simulink model "Clutchless_P2_Parallel_ETE"  (R2017b)
settings: Solver=FixedStepAuto  StartTime=0.0  StopTime=length(Speed)  FixedStep=0.01  MaxStep=0.01  RelTol=1e-3  EnableMultiTasking=on
PostLoadFcn:
  | , if any(exist('dsrtsu_mdlpostloadfcn', 'file') == [2, 3, 6]), try dsrtsu_mdlpostloadfcn('Execute', bdroot); catch fprintf('Error in PostLoadFcn (dsrtsu_mdlpostloadfcn) for model "%s":\n %s\n', bdroot, lasterr); end, end,
undefined symbols (not defined in the file): ABSEnable, Actuators, air, APP1_OOR, APP2_OOR, APP_Mismatch, Brk_Flt, cal, ClutchEngag, Clutchless_HSC_ETE, CS_On_Control, Driver, eng, Engine, EngOverTemp, ENGTRQ_MSMCH_Degraded_CP, ENGTRQ_MSMCH_ErrCritical_CP, ENGTRQ_MSMCH_LimpHome_CP, EngTrqMismatch, env, ess, ESSOverTemp, gb, KeyPos_Flt, KeyPosition, lib_Actuators, lib_Clutchless_HSC_ETE, lib_Driver, lib_EMachine_2017a, lib_Sensors_2017a, LossCAN, Machine, max_vehicle_rad_air_flow, MCUOverTemp, mot, MotDirMismatch, MotOverTemp, MotTrqMismatch, mph2ms, PRNDL_Flt, RegenBrkDisable, RegenFault, Sensors, ShiftLeverPosition, Speed, SW_CS_ON, SW_Engine_ON, t_amb, time, tloop
libraries: simulink x97, Pneumatic_lib x11, nesl_utility x9, EC2_libraries x7, powerlib_meascontrol x2, CalculationGallon x1, lib_Chassis x1, lib_DCDC x1, lib_Differential x1, lib_HVESS x1, fl_lib x1, lib_OBC x1
(part 7 of 9)

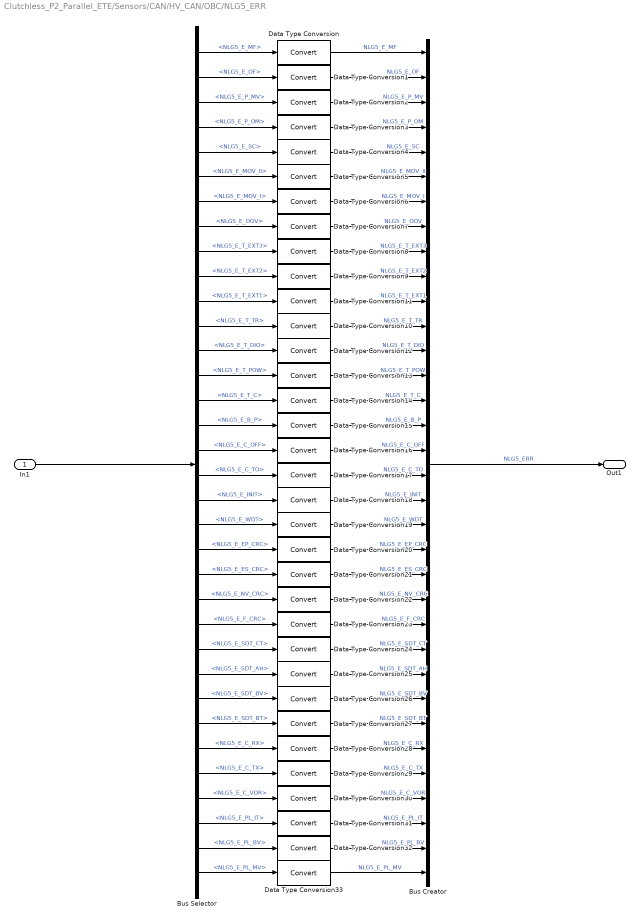
== system Clutchless_P2_Parallel_ETE/Sensors/CAN/HV_CAN/OBC/NLG5_ERR ==
  In1 : Inport
  Bus Creator : BusCreator  Inputs=34
  Bus Selector : BusSelector  OutputSignals=NLG5_E_MF,NLG5_E_OF,NLG5_E_P_MV,NLG5_E_P_OM,NLG5_E_SC,NLG5_E_MOV_II,NLG5_E_MOV_I,NLG5_E_OOV,NLG5_E_T_EXT3,NLG5_E_T_EXT2,NLG5_E_T_EXT1,NLG5_E_T_TR,NLG5_E_T_DIO,NLG5_E_T_POW,NLG5_E_T_C,NLG5_E_B_P,NLG5_E_C_OFF,NLG5_E_C_TO,NLG5_E_INIT,NLG5_E_WDT,NLG5_E_EP_CRC,NLG5_E_ES_CRC,NLG5_E_NV_CRC,NLG5_E_F_CRC,NLG5_E_SDT_CT,NLG5_E_SDT_AH,NLG5_E_SDT_BV,NLG5_E_SDT_BT,NLG5_E_C_RX,NLG5_E_C_TX,NLG5_E_C_VOR,NLG5_E_PL_IT,NLG5_E_PL_BV,NLG5_E_PL_MV
  Data Type Conversion{,1..33} (34 alike) : DataTypeConversion
  Out1 : Outport
  wires:
  Data Type Conversion4/1 -> Bus Creator/5  "NLG5_E_SC"
  Bus Selector/5 -> Data Type Conversion4/1  "<NLG5_E_SC>"
  In1/1 -> Bus Selector/1
  Bus Selector/1 -> Data Type Conversion/1  "<NLG5_E_MF>"
  Bus Selector/2 -> Data Type Conversion1/1  "<NLG5_E_OF>"
  Bus Selector/3 -> Data Type Conversion2/1  "<NLG5_E_P_MV>"
  Bus Selector/4 -> Data Type Conversion3/1  "<NLG5_E_P_OM>"
  Data Type Conversion/1 -> Bus Creator/1  "NLG5_E_MF"
  Data Type Conversion1/1 -> Bus Creator/2  "NLG5_E_OF"
  Data Type Conversion2/1 -> Bus Creator/3  "NLG5_E_P_MV"
  Data Type Conversion3/1 -> Bus Creator/4  "NLG5_E_P_OM"
  Bus Creator/1 -> Out1/1  "NLG5_ERR"
  Bus Selector/6 -> Data Type Conversion5/1  "<NLG5_E_MOV_II>"
  Bus Selector/34 -> Data Type Conversion33/1  "<NLG5_E_PL_MV>"
  Bus Selector/33 -> Data Type Conversion32/1  "<NLG5_E_PL_BV>"
  Bus Selector/32 -> Data Type Conversion31/1  "<NLG5_E_PL_IT>"
  Bus Selector/31 -> Data Type Conversion30/1  "<NLG5_E_C_VOR>"
  Bus Selector/30 -> Data Type Conversion29/1  "<NLG5_E_C_TX>"
  Bus Selector/29 -> Data Type Conversion28/1  "<NLG5_E_C_RX>"
  Bus Selector/28 -> Data Type Conversion27/1  "<NLG5_E_SDT_BT>"
  Bus Selector/27 -> Data Type Conversion26/1  "<NLG5_E_SDT_BV>"
  Bus Selector/7 -> Data Type Conversion6/1  "<NLG5_E_MOV_I>"
  Bus Selector/8 -> Data Type Conversion7/1  "<NLG5_E_OOV>"
  Bus Selector/9 -> Data Type Conversion8/1  "<NLG5_E_T_EXT3>"
  Bus Selector/10 -> Data Type Conversion9/1  "<NLG5_E_T_EXT2>"
  Bus Selector/11 -> Data Type Conversion11/1  "<NLG5_E_T_EXT1>"
  Bus Selector/12 -> Data Type Conversion10/1  "<NLG5_E_T_TR>"
  Bus Selector/13 -> Data Type Conversion12/1  "<NLG5_E_T_DIO>"
  Bus Selector/14 -> Data Type Conversion13/1  "<NLG5_E_T_POW>"
  Bus Selector/15 -> Data Type Conversion14/1  "<NLG5_E_T_C>"
  Bus Selector/16 -> Data Type Conversion15/1  "<NLG5_E_B_P>"
  Bus Selector/17 -> Data Type Conversion16/1  "<NLG5_E_C_OFF>"
  Bus Selector/18 -> Data Type Conversion17/1  "<NLG5_E_C_TO>"
  Bus Selector/19 -> Data Type Conversion18/1  "<NLG5_E_INIT>"
  Bus Selector/20 -> Data Type Conversion19/1  "<NLG5_E_WDT>"
  Bus Selector/21 -> Data Type Conversion20/1  "<NLG5_E_EP_CRC>"
  Bus Selector/22 -> Data Type Conversion21/1  "<NLG5_E_ES_CRC>"
  Bus Selector/23 -> Data Type Conversion22/1  "<NLG5_E_NV_CRC>"
  Bus Selector/24 -> Data Type Conversion23/1  "<NLG5_E_F_CRC>"
  Bus Selector/25 -> Data Type Conversion24/1  "<NLG5_E_SDT_CT>"
  Bus Selector/26 -> Data Type Conversion25/1  "<NLG5_E_SDT_AH>"
  Data Type Conversion5/1 -> Bus Creator/6  "NLG5_E_MOV_II"
  Data Type Conversion6/1 -> Bus Creator/7  "NLG5_E_MOV_I"
  Data Type Conversion7/1 -> Bus Creator/8  "NLG5_E_OOV"
  Data Type Conversion8/1 -> Bus Creator/9  "NLG5_E_T_EXT3"
  Data Type Conversion9/1 -> Bus Creator/10  "NLG5_E_T_EXT2"
  Data Type Conversion11/1 -> Bus Creator/11  "NLG5_E_T_EXT1"
  Data Type Conversion10/1 -> Bus Creator/12  "NLG5_E_T_TR"
  Data Type Conversion12/1 -> Bus Creator/13  "NLG5_E_T_DIO"
  Data Type Conversion13/1 -> Bus Creator/14  "NLG5_E_T_POW"
  Data Type Conversion14/1 -> Bus Creator/15  "NLG5_E_T_C"
  Data Type Conversion15/1 -> Bus Creator/16  "NLG5_E_B_P"
  Data Type Conversion16/1 -> Bus Creator/17  "NLG5_E_C_OFF"
  Data Type Conversion17/1 -> Bus Creator/18  "NLG5_E_C_TO"
  Data Type Conversion18/1 -> Bus Creator/19  "NLG5_E_INIT"
  Data Type Conversion19/1 -> Bus Creator/20  "NLG5_E_WDT"
  Data Type Conversion20/1 -> Bus Creator/21  "NLG5_E_EP_CRC"
  Data Type Conversion21/1 -> Bus Creator/22  "NLG5_E_ES_CRC"
  Data Type Conversion22/1 -> Bus Creator/23  "NLG5_E_NV_CRC"
  Data Type Conversion23/1 -> Bus Creator/24  "NLG5_E_F_CRC"
  Data Type Conversion24/1 -> Bus Creator/25  "NLG5_E_SDT_CT"
  Data Type Conversion25/1 -> Bus Creator/26  "NLG5_E_SDT_AH"
  Data Type Conversion26/1 -> Bus Creator/27  "NLG5_E_SDT_BV"
  Data Type Conversion27/1 -> Bus Creator/28  "NLG5_E_SDT_BT"
  Data Type Conversion28/1 -> Bus Creator/29  "NLG5_E_C_RX"
  Data Type Conversion29/1 -> Bus Creator/30  "NLG5_E_C_TX"
  Data Type Conversion30/1 -> Bus Creator/31  "NLG5_E_C_VOR"
  Data Type Conversion31/1 -> Bus Creator/32  "NLG5_E_PL_IT"
  Data Type Conversion32/1 -> Bus Creator/33  "NLG5_E_PL_BV"
  Data Type Conversion33/1 -> Bus Creator/34  "NLG5_E_PL_MV"

== system Clutchless_P2_Parallel_ETE/Sensors/CAN/HV_CAN/OBC/NLG5_ST ==
  In1 : Inport
  Bus Creator : BusCreator  Inputs=24
  Bus Selector : BusSelector  OutputSignals=NLG5_S_CP_DT,NLG5_S_UM_II,NLG5_S_UM_I,NLG5_S_EUM,NLG5_S_FAN,NLG5_S_WAR,NLG5_S_ERR,NLG5_S_HE,NLG5_S_L_PMAX,NLG5_S_L_CP,NLG5_S_L_PI,NLG5_S_L_MC,NLG5_S_L_OC,NLG5_S_L_OV,NLG5_S_BPD_II,NLG5_S_BPD_I,NLG5_S_L_T_BATT,NLG5_S_L_T_TR,NLG5_S_L_T_DIO,NLG5_S_L_T_POW,NLG5_S_L_T_CPRIM,NLG5_S_L_MO_MAX,NLG5_S_L_OC_MAX,NLG5_S_L_MC_MAX
  Data Type Conversion{,1..23} (24 alike) : DataTypeConversion
  Out1 : Outport
  wires:
  Data Type Conversion4/1 -> Bus Creator/5  "NLG5_S_FAN"
  Bus Selector/5 -> Data Type Conversion4/1  "<NLG5_S_FAN>"
  In1/1 -> Bus Selector/1
  Bus Selector/1 -> Data Type Conversion/1  "<NLG5_S_CP_DT>"
  Bus Selector/2 -> Data Type Conversion1/1  "<NLG5_S_UM_II>"
  Bus Selector/3 -> Data Type Conversion2/1  "<NLG5_S_UM_I>"
  Bus Selector/4 -> Data Type Conversion3/1  "<NLG5_S_EUM>"
  Data Type Conversion/1 -> Bus Creator/1  "NLG5_S_CP_DT"
  Data Type Conversion1/1 -> Bus Creator/2  "NLG5_S_UM_II"
  Data Type Conversion2/1 -> Bus Creator/3  "NLG5_S_UM_I"
  Data Type Conversion3/1 -> Bus Creator/4  "NLG5_S_EUM"
  Bus Creator/1 -> Out1/1  "NLG5_ST"
  Bus Selector/6 -> Data Type Conversion5/1  "<NLG5_S_WAR>"
  Bus Selector/7 -> Data Type Conversion6/1  "<NLG5_S_ERR>"
  Bus Selector/8 -> Data Type Conversion7/1  "<NLG5_S_HE>"
  Bus Selector/9 -> Data Type Conversion8/1  "<NLG5_S_L_PMAX>"
  Bus Selector/10 -> Data Type Conversion9/1  "<NLG5_S_L_CP>"
  Bus Selector/11 -> Data Type Conversion10/1  "<NLG5_S_L_PI>"
  Bus Selector/12 -> Data Type Conversion11/1  "<NLG5_S_L_MC>"
  Bus Selector/13 -> Data Type Conversion12/1  "<NLG5_S_L_OC>"
  Bus Selector/14 -> Data Type Conversion13/1  "<NLG5_S_L_OV>"
  Bus Selector/15 -> Data Type Conversion14/1  "<NLG5_S_BPD_II>"
  Bus Selector/16 -> Data Type Conversion15/1  "<NLG5_S_BPD_I>"
  Bus Selector/17 -> Data Type Conversion16/1  "<NLG5_S_L_T_BATT>"
  Bus Selector/18 -> Data Type Conversion17/1  "<NLG5_S_L_T_TR>"
  Bus Selector/19 -> Data Type Conversion18/1  "<NLG5_S_L_T_DIO>"
  Bus Selector/20 -> Data Type Conversion19/1  "<NLG5_S_L_T_POW>"
  Bus Selector/21 -> Data Type Conversion20/1  "<NLG5_S_L_T_CPRIM>"
  Bus Selector/22 -> Data Type Conversion21/1  "<NLG5_S_L_MO_MAX>"
  Bus Selector/23 -> Data Type Conversion22/1  "<NLG5_S_L_OC_MAX>"
  Bus Selector/24 -> Data Type Conversion23/1  "<NLG5_S_L_MC_MAX>"
  Data Type Conversion5/1 -> Bus Creator/6  "NLG5_S_WAR"
  Data Type Conversion7/1 -> Bus Creator/8  "NLG5_S_HE"
  Data Type Conversion6/1 -> Bus Creator/7  "NLG5_S_ERR"
  Data Type Conversion8/1 -> Bus Creator/9  "NLG5_S_L_PMAX"
  Data Type Conversion9/1 -> Bus Creator/10  "NLG5_S_L_CP"
  Data Type Conversion10/1 -> Bus Creator/11  "NLG5__S_L_PI"
  Data Type Conversion11/1 -> Bus Creator/12  "NLG5_S_L_MC"
  Data Type Conversion12/1 -> Bus Creator/13  "NLG5_S_L_OC"
  Data Type Conversion13/1 -> Bus Creator/14  "NLG5_S_L_OV"
  Data Type Conversion14/1 -> Bus Creator/15  "NLG5_S_BPD_II"
  Data Type Conversion15/1 -> Bus Creator/16  "NLG5_S_BPD_I"
  Data Type Conversion16/1 -> Bus Creator/17  "NLG5_S_L_T_BATT"
  Data Type Conversion17/1 -> Bus Creator/18  "NLG5_S_L_T_TR"
  Data Type Conversion18/1 -> Bus Creator/19  "NLG5_S_L_T_DIO"
  Data Type Conversion19/1 -> Bus Creator/20  "NLG5_S_L_T_POW"
  Data Type Conversion20/1 -> Bus Creator/21  "NLG5_S_L_T_CPRM"
  Data Type Conversion21/1 -> Bus Creator/22  "NLG5_S_L_MO_MAX"
  Data Type Conversion22/1 -> Bus Creator/23  "NLG5_S_L_OC_MAX"
  Data Type Conversion23/1 -> Bus Creator/24  "NLG5_S_L_MC_MAX"

== system Clutchless_P2_Parallel_ETE/Sensors/CAN/HV_CAN/OBC/NLG5_TEMP ==
  In1 : Inport
  Bus Creator : BusCreator  Inputs=4
  Bus Selector : BusSelector  OutputSignals=NLG5_P_TMP,NLG5_TMP_EXT1,NLG5_TMP_EXT2,NLG5_TMP_EXT3
  Data Type Conversion{,1..3} (4 alike) : DataTypeConversion
  Out1 : Outport
  wires:
  In1/1 -> Bus Selector/1
  Bus Selector/1 -> Data Type Conversion/1  "<NLG5_P_TMP>"
  Bus Selector/2 -> Data Type Conversion1/1  "<NLG5_TMP_EXT1>"
  Bus Selector/3 -> Data Type Conversion2/1  "<NLG5_TMP_EXT2>"
  Bus Selector/4 -> Data Type Conversion3/1  "<NLG5_TMP_EXT3>"
  Data Type Conversion/1 -> Bus Creator/1  "NLG5_P_TMP"
  Data Type Conversion1/1 -> Bus Creator/2  "NLG5_TMP_EXT1"
  Data Type Conversion2/1 -> Bus Creator/3  "NLG5_TMP_EXT2"
  Data Type Conversion3/1 -> Bus Creator/4  "NLG5_TMP_EXT3"
  Bus Creator/1 -> Out1/1  "NLG5_TEMP"

== system Clutchless_P2_Parallel_ETE/Sensors/CAN/VEH_CAN/BCM/PPEI_Brake_Apply_Status ==
  In1 : Inport
  Out1 : Outport
  wires:
  In1/1 -> Out1/1  "BrkPdlPos"

== system Clutchless_P2_Parallel_ETE/Sensors/CAN/VEH_CAN/BCM/PPEI_Platfrom_General_Status ==
  In1 : Inport
  Out1 : Outport
  wires:
  In1/1 -> Out1/1  "SysPwrMd"

== system Clutchless_P2_Parallel_ETE/Sensors/CAN/VEH_CAN/EBCM/PPEI_Chassis_General_Status_1 ==
  In1 : Inport
  Out1 : Outport
  wires:
  In1/1 -> Out1/1  "BrkPdlDrvAppPrsDetcd"

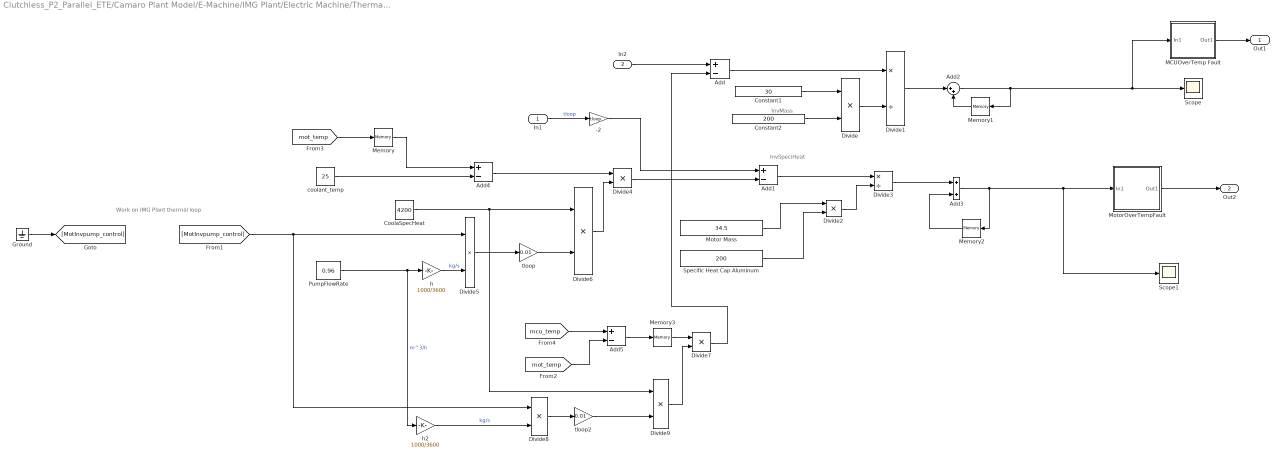
== system Clutchless_P2_Parallel_ETE/Camaro Plant Model/E-Machine/IMG Plant/Electric Machine/Thermal1/MotInv_loop ==
  note: Work on IMG Plant thermal loop
  note: InvMass
  note: InvSpeciHeat
  In1 : Inport
  In2 : Inport  Port=2
  -2 : Gain  Gain=tloop
  Add{,1,4..5} (4 alike) : Sum  Inputs=+-
  Add2 : Sum  Inputs=|++
  Add3 : Sum
  Constant1 : Constant  Value=30
  Constant2 : Constant  Value=200
  CoolaSpecHeat : Constant  Value=4200
  Divide{,2,4..9} (8 alike) : Product  Inputs=**
  Divide1 : Product  Inputs=*/
  Divide3 : Product  Inputs=*/
  Ground : Ground
  MCUOverTemp Fault : Subsystem
  Memory : Memory
  Memory1 : Memory  InitialCondition=25
  Memory2 : Memory  InitialCondition=25
  Memory3 : Memory
  Motor Mass : Constant  Value=34.5
  MotorOverTempFault : Subsystem
  PumpFlowRate : Constant  Value=0.96
  Scope : Scope
  Scope1 : Scope
  Specific Heat Cap Aluminum : Constant  Value=200
  coolant_temp : Constant  Value=25
  h : Gain  Gain=1000/3600
  h2 : Gain  Gain=1000/3600
  tloop : Gain  Gain=0.01
  tloop2 : Gain  Gain=0.01
  Out1 : Outport
  Out2 : Outport  Port=2
  wires:
  [MotInvpump_control] -> Divide8/1, Divide5/1
  -2/1 -> Add1/1
  In2/1 -> Add/1
  In1/1 -> -2/1  "tloop"
  [mot_temp] -> Add5/2
  [mcu_temp] -> Add5/1
  [mot_temp] -> Memory/1
  MotorOverTempFault/1(Out1) -> Out2/1
  MCUOverTemp Fault/1(Out1) -> Out1/1
  Memory3/1 -> Divide7/1
  Add5/1 -> Memory3/1
  Divide4/1 -> Add1/2
  tloop2/1 -> Divide9/2
  Divide8/1 -> tloop2/1
  Divide9/1 -> Divide7/2
  h2/1 -> Divide8/2  "kg/s"
  PumpFlowRate/1 -> h2/1, h/1  "m^3/h"
  CoolaSpecHeat/1 -> Divide9/1, Divide6/1
  tloop/1 -> Divide6/2
  h/1 -> Divide5/2  "kg/s"
  Divide7/1 -> Add/2
  Divide1/1 -> Add2/1
  Motor Mass/1 -> Divide2/1
  Constant2/1 -> Divide/2
  Divide2/1 -> Divide3/2
  Add2/1 -> Memory1/1, Scope/1, MCUOverTemp Fault/1(In1)
  Divide5/1 -> tloop/1
  Divide3/1 -> Add3/1
  Divide6/1 -> Divide4/2
  Add3/1 -> Memory2/1, MotorOverTempFault/1(In1), Scope1/1
  Add4/1 -> Divide4/1
  Memory2/1 -> Add3/2
  Add/1 -> Divide1/1
  Constant1/1 -> Divide/1
  Specific Heat Cap Aluminum/1 -> Divide2/2
  Divide/1 -> Divide1/2
  coolant_temp/1 -> Add4/2
  Memory1/1 -> Add2/2
  Add1/1 -> Divide3/1
  Memory/1 -> Add4/1
  Ground/1 -> [MotInvpump_control]

== system Clutchless_P2_Parallel_ETE/Camaro Plant Model/E-Machine/IMG Plant/Electric Machine/Thermal1/Motor Thermal ==
  In1 : Inport
  Add1 : Sum  Inputs=+-
  Add2 : Sum
  Divide : Product  Inputs=*/
  Lower Limit : Subsystem  mask{Lolimit=t_amb+20}
      mask prompts: Lolimit "Lower Limit"
  Memory1 : Memory
  Motor Mass : Constant  Value=mot.plant.init.motor_mass
  Product : Product  RndMeth=Zero
  "Pump " : Constant  Value=0
  Specific Heat Cap Aluminum : Constant  Value=mot.plant.init.specific_heat
  tloop : Gain  Gain=tloop
  Out1 : Outport
  wires:
  Add1/1 -> tloop/1
  In1/1 -> Add1/1
  "Pump "/1 -> Add1/2
  Motor Mass/1 -> Product/1  "kg"
  tloop/1 -> Divide/1  "J"
  Divide/1 -> Add2/1
  Lower Limit/1(Out1) -> Memory1/1, Out1/1
  Add2/1 -> Lower Limit/1(In1)
  Memory1/1 -> Add2/2
  Product/1 -> Divide/2
  Specific Heat Cap Aluminum/1 -> Product/2  "J/kg*K"

== system Clutchless_P2_Parallel_ETE/Camaro Plant Model/E-Machine/IMG Plant/Electric Machine/Torque Calculation1/electric machine filter ==
  trq : Inport
  Interval Test : simulink/Logic and Bit Operations/Interval Test  IntervalClosedRight=on  uplimit=0.5  IntervalClosedLeft=on  lowlimit=-0.5  OutDataTypeStr=boolean
  Switch : Switch  Threshold=0.5
  electric machine time response : TransferFcn  Denominator=[mot.plant.init.time_response 1]
  filtered : Outport
  wires:
  Switch/1 -> filtered/1
  trq/1 -> Switch/1, electric machine time response/1, Interval Test/1
  Interval Test/1 -> Switch/2
  electric machine time response/1 -> Switch/3

== system Clutchless_P2_Parallel_ETE/Camaro Plant Model/E-Machine/IMG Plant/Electric Machine/Torque Calculation1/max torque  ==
  cmd : Inport
  speed : Inport  Port=2
  Memory : Memory
  Peak trq max - Motoring : Lookup  InputValues=mot.plant.init.regen.trq_max.idx1_spd  Table=mot.plant.init.motor.trq_max.map  LookUpMeth=Interpolation-Use End Values  SaturateOnIntegerOverflow=on
  Peak trq max - Regen : Lookup  InputValues=mot.plant.init.regen.trq_max.idx1_spd  Table=mot.plant.init.regen.trq_max.map  LookUpMeth=Interpolation-Use End Values  SaturateOnIntegerOverflow=on
  Switch1 : Switch  SaturateOnIntegerOverflow=on
  rad/s  to RPM : Gain  Gain=30/pi
  max torque : Outport
  wires:
  Peak trq max - Regen/1 -> Switch1/3
  rad/s  to RPM/1 -> Memory/1
  Memory/1 -> Peak trq max - Regen/1, Peak trq max - Motoring/1
  Switch1/1 -> max torque/1
  cmd/1 -> Switch1/2
  speed/1 -> rad/s  to RPM/1
  Peak trq max - Motoring/1 -> Switch1/1

== system Clutchless_P2_Parallel_ETE/Camaro Plant Model/E-Machine/IMG Plant2/Thermal/Motor Thermal/Lower Limit ==
  In1 : Inport
  Constant3 : Constant  Value=Lolimit
  MinMax : MinMax  Function=max  Inputs=2
  Out1 : Outport
  wires:
  MinMax/1 -> Out1/1
  Constant3/1 -> MinMax/2
  In1/1 -> MinMax/1

== system Clutchless_P2_Parallel_ETE/Camaro Plant Model/E-Machine/IMG Plant2/Thermal1/MotInv_loop/MCUOverTemp Fault ==
  In1 : Inport
  Gain : Gain  Gain=3
  Switch : Switch  Threshold=1
  Out1 : Outport
  wires:
  Switch/1 -> Out1/1
  Gain/1 -> Switch/1
  [MCUOverTemp] -> Switch/2
  In1/1 -> Gain/1, Switch/3

== system Clutchless_P2_Parallel_ETE/Camaro Plant Model/E-Machine/IMG Plant2/Thermal1/MotInv_loop/MotorOverTempFault ==
  In1 : Inport
  Gain : Gain  Gain=2
  Switch1 : Switch  Threshold=1
  Out1 : Outport
  wires:
  Switch1/1 -> Out1/1
  Gain/1 -> Switch1/1
  [MotOverTemp] -> Switch1/2
  In1/1 -> Switch1/3, Gain/1

== system Clutchless_P2_Parallel_ETE/Camaro Plant Model/E-Machine/IMG Plant2/Thermal1/Motor Thermal/Lower Limit ==
  In1 : Inport
  Constant3 : Constant  Value=Lolimit
  MinMax : MinMax  Function=max  Inputs=2
  Out1 : Outport
  wires:
  MinMax/1 -> Out1/1
  Constant3/1 -> MinMax/2
  In1/1 -> MinMax/1

== system Clutchless_P2_Parallel_ETE/Camaro Plant Model/E-Machine/Soft MCU/Torque Calculation1/max torque /Divide by zero ==
  In1 : Inport
  Compare To Constant : simulink/Logic and Bit Operations/Compare To Constant  relop===  const=0  OutDataTypeStr=boolean
  Constant1 : Constant
  Switch2 : Switch  Criteria=u2 > Threshold
  Out1 : Outport
  wires:
  Constant1/1 -> Switch2/1
  Compare To Constant/1 -> Switch2/2
  In1/1 -> Switch2/3, Compare To Constant/1
  Switch2/1 -> Out1/1

== system Clutchless_P2_Parallel_ETE/Camaro Plant Model/E-Machine/Soft MCU/Torque Calculation1/max torque /Heat index ==
  note: Heat index calculation
  cont torque : Inport
  torque : Inport  Port=2
  Abs : Abs  SaturateOnIntegerOverflow=on
  Divide : Subsystem  mask(Divide){}
      mask Display: disp('Divide')
  Heat Energy Factor : Integrator  InitialCondition=-0.3  LimitOutput=on  UpperSaturationLimit=1  LowerSaturationLimit=-0.3
  Heating Constant : Gain  Gain=0.3/mot.plant.init.t_max_trq  SaturateOnIntegerOverflow=on  OutDataTypeStr=Inherit: Same as input  ParamDataTypeStr=Inherit: Same as input
  Saturation : Saturate  UpperLimit=1  LowerLimit=0
  Sum : Sum  Inputs=+-  SaturateOnIntegerOverflow=on  InputSameDT=on  OutDataTypeStr=Inherit: Same as first input
  motor inertia (Nms^2\rad)5 : Constant
  Heat index : Outport
  wires:
  cont torque/1 -> Divide/2(denominator)
  Abs/1 -> Sum/1
  Saturation/1 -> Heat index/1
  motor inertia (Nms^2\rad)5/1 -> Sum/2
  Divide/1(quotient) -> Abs/1
  Sum/1 -> Heating Constant/1
  Heating Constant/1 -> Heat Energy Factor/1
  Heat Energy Factor/1 -> Saturation/1
  torque/1 -> Divide/1(numerator)

== system Clutchless_P2_Parallel_ETE/Camaro Plant Model/E-Machine/Soft MCU/Torque Calculation2/max torque /Divide by zero ==
  In1 : Inport
  Compare To Constant : simulink/Logic and Bit Operations/Compare To Constant  relop===  const=0  OutDataTypeStr=boolean
  Constant1 : Constant
  Switch2 : Switch  Criteria=u2 > Threshold
  Out1 : Outport
  wires:
  Constant1/1 -> Switch2/1
  Compare To Constant/1 -> Switch2/2
  In1/1 -> Switch2/3, Compare To Constant/1
  Switch2/1 -> Out1/1

== system Clutchless_P2_Parallel_ETE/Camaro Plant Model/E-Machine/Soft MCU/Torque Calculation2/max torque /Heat index ==
  note: Heat index calculation
  cont torque : Inport
  torque : Inport  Port=2
  Abs : Abs  SaturateOnIntegerOverflow=on
  Divide : Subsystem  mask(Divide){}
      mask Display: disp('Divide')
  Heat Energy Factor : Integrator  InitialCondition=-0.3  LimitOutput=on  UpperSaturationLimit=1  LowerSaturationLimit=-0.3
  Heating Constant : Gain  Gain=0.3/mot.plant.init.t_max_trq  SaturateOnIntegerOverflow=on  OutDataTypeStr=Inherit: Same as input  ParamDataTypeStr=Inherit: Same as input
  Saturation : Saturate  UpperLimit=1  LowerLimit=0
  Sum : Sum  Inputs=+-  SaturateOnIntegerOverflow=on  InputSameDT=on  OutDataTypeStr=Inherit: Same as first input
  motor inertia (Nms^2\rad)5 : Constant
  Heat index : Outport
  wires:
  cont torque/1 -> Divide/2(denominator)
  Abs/1 -> Sum/1
  Saturation/1 -> Heat index/1
  motor inertia (Nms^2\rad)5/1 -> Sum/2
  Divide/1(quotient) -> Abs/1
  Sum/1 -> Heating Constant/1
  Heating Constant/1 -> Heat Energy Factor/1
  Heat Energy Factor/1 -> Saturation/1
  torque/1 -> Divide/1(numerator)

== system Clutchless_P2_Parallel_ETE/Camaro Plant Model/ICE Simple1/Engine Plant Modified/Core Engine/Core Engine1/Upstream States ==
  K Converter : nesl_utility/PS-Simulink Converter  PhysicalDomain=network_engine_domain  SubClassName=ps_output  LeftPortType=input  RightPortType=output  PseudoPeriodic=off  Frequencies=[]  Unit=K  AffineConversion=off
  Pa Converter : nesl_utility/PS-Simulink Converter  PhysicalDomain=network_engine_domain  SubClassName=ps_output  LeftPortType=input  RightPortType=output  PseudoPeriodic=off  Frequencies=[]  Unit=Pa  AffineConversion=off
  Pneumatic Absolute Reference : Pneumatic_lib/Pneumatic Elements/Pneumatic Absolute Reference
  Pneumatic Pressure & Temperature Sensor : Pneumatic_lib/Pneumatic Sensors/Pneumatic Pressure & Temperature Sensor
  A : PMIOPort  Port=1  Side=Left
  P (Pa) : Outport
  T (K) : Outport  Port=2
  wires:
  Pa Converter/1 -> P (Pa)/1
  K Converter/1 -> T (K)/1
  connections:
  Pneumatic Pressure & Temperature Sensor/RConn1 -- Pneumatic Absolute Reference/LConn1
  Pneumatic Pressure & Temperature Sensor/LConn1 -- A/RConn1
  K Converter/LConn1 -- Pneumatic Pressure & Temperature Sensor/RConn3
  Pneumatic Pressure & Temperature Sensor/RConn2 -- Pa Converter/LConn1

== system Clutchless_P2_Parallel_ETE/Camaro Plant Model/ICE Simple1/Engine Plant Modified/Core Engine/EngEfficiency1/Divide by Zero Fix ==
  Multiply : Inport
  Divide : Inport  Port=2
  Compare To Zero : simulink/Logic and Bit Operations/Compare To Zero  relop===  OutDataTypeStr=boolean
  Constant1 : Constant  Value=0
  Constant2 : Constant
  Product2 : Product  Inputs=/*  SaturateOnIntegerOverflow=on  InputSameDT=on  OutDataTypeStr=Inherit: Same as first input
  Switch : Switch  Threshold=1
  Switch1 : Switch  Threshold=1
  Output : Outport
  wires:
  Multiply/1 -> Product2/2
  Switch1/1 -> Output/1
  Constant1/1 -> Switch1/1
  Product2/1 -> Switch1/3
  Switch/1 -> Product2/1
  Divide/1 -> Switch/3, Compare To Zero/1
  Constant2/1 -> Switch/1
  Compare To Zero/1 -> Switch1/2, Switch/2

== system Clutchless_P2_Parallel_ETE/Camaro Plant Model/ICE Simple1/Engine Plant Modified/Core Engine/Intake Manifold1/Node Potential Sensor ==
  K Converter : nesl_utility/PS-Simulink Converter  PhysicalDomain=network_engine_domain  SubClassName=ps_output  LeftPortType=input  RightPortType=output  PseudoPeriodic=off  Frequencies=[]  Unit=K  AffineConversion=off
  K to C : Fcn  Expr=u(1)-273.15
  Pa Converter : nesl_utility/PS-Simulink Converter  PhysicalDomain=network_engine_domain  SubClassName=ps_output  LeftPortType=input  RightPortType=output  PseudoPeriodic=off  Frequencies=[]  Unit=Pa  AffineConversion=off
  Pa to KPa : Gain  Gain=0.001
  Pneumatic Absolute Reference : Pneumatic_lib/Pneumatic Elements/Pneumatic Absolute Reference
  Pneumatic Pressure & Temperature Sensor : Pneumatic_lib/Pneumatic Sensors/Pneumatic Pressure & Temperature Sensor
  A : PMIOPort  Port=1  Side=Left
  P (KPa) : Outport
  T (C) : Outport  Port=2
  wires:
  Pa Converter/1 -> Pa to KPa/1
  K Converter/1 -> K to C/1
  K to C/1 -> T (C)/1
  Pa to KPa/1 -> P (KPa)/1
  connections:
  Pneumatic Pressure & Temperature Sensor/RConn1 -- Pneumatic Absolute Reference/LConn1
  Pneumatic Pressure & Temperature Sensor/LConn1 -- A/RConn1
  K Converter/LConn1 -- Pneumatic Pressure & Temperature Sensor/RConn3
  Pneumatic Pressure & Temperature Sensor/RConn2 -- Pa Converter/LConn1

== system Clutchless_P2_Parallel_ETE/Clutchless_HSC_ETE/HSC/Camaro Fault Detection/Component Diagnostic/Engine Component Diagnostic/Override  engTrqCmd ==
  note: This subsystem is used to override the model value of a signal to a constant value
  note: Override Switch Subsystem
  In1 : Inport
  Constant : Constant  Value=50
  Multiport Switch : MultiPortSwitch  DataPortOrder=Zero-based contiguous  Inputs=2  zeroidx=on
  Signal Override Switch 0 = Use Model 1 = Use Constant : Constant
  Out1 : Outport
  wires:
  Signal Override Switch 0 = Use Model 1 = Use Constant/1 -> Multiport Switch/1
  In1/1 -> Multiport Switch/2
  Multiport Switch/1 -> Out1/1
  Constant/1 -> Multiport Switch/3

== system Clutchless_P2_Parallel_ETE/Clutchless_HSC_ETE/HSC/Camaro Fault Detection/Component Diagnostic/Engine Component Diagnostic/TorqMismatch Detection ==
  In1 : Inport
  In2 : Inport  Port=2
  In3 : Inport  Port=3
  Abs : Abs
  Add : Sum  Inputs=+-
  Bus Creator : BusCreator  Inputs=3
  Constant : Constant  Value=cal.ENGTRQ_MSMCH.ErrCritical_CP
  Constant1 : Constant  Value=50
  Constant2 : Constant  Value=cal.ENGTRQ_MSMCH.Degraded_CP
  Constant3 : Constant  Value=cal.ENGTRQ_MSMCH.LimpHome_CP
  Constant4 : Constant  Value=0
  Constant5 : Constant  Value=0
  Constant6 : Constant  Value=0
  Data Type Conversion : DataTypeConversion  OutDataTypeStr=boolean
  Data Type Conversion1 : DataTypeConversion  OutDataTypeStr=boolean
  Data Type Conversion2 : DataTypeConversion  OutDataTypeStr=boolean
  Relational Operator : RelationalOperator  OutDataTypeStr=boolean  RndMeth=Nearest
  Relational Operator1 : RelationalOperator  Operator=>  OutDataTypeStr=boolean  RndMeth=Nearest
  Relational Operator2 : RelationalOperator  Operator=>  OutDataTypeStr=boolean  RndMeth=Nearest
  Switch : Switch  Threshold=1
  Terminator{,1..3} (4 alike) : Terminator
  Unit Delay : UnitDelay  Commented=through  SampleTime=-1
  Unit Delay1 : UnitDelay  Commented=through  SampleTime=-1
  "Zero " : Constant  Value=0
  Eng_Torque_Mismch : Outport
  wires:
  Constant1/1 -> Terminator3/1
  In1/1 -> Unit Delay/1
  In2/1 -> Unit Delay1/1
  "Zero "/1 -> Switch/3
  In3/1 -> Switch/2
  Unit Delay/1 -> Add/1
  Constant/1 -> Relational Operator/2
  Add/1 -> Abs/1
  Relational Operator/1 -> Switch/1
  Switch/1 -> Relational Operator2/1, Relational Operator1/1, Terminator/1  "Eng_Torque_Mismch_Critical"
  Constant2/1 -> Relational Operator1/2
  Constant3/1 -> Relational Operator2/2
  Relational Operator1/1 -> Terminator1/1  "Eng_Torque_Mismch_Degrad"
  Relational Operator2/1 -> Terminator2/1  "Eng_Torque_Mismch_Limp"
  Bus Creator/1 -> Eng_Torque_Mismch/1
  Unit Delay1/1 -> Add/2
  Abs/1 -> Relational Operator/1
  Constant4/1 -> Data Type Conversion/1  "Eng_Torque_Mismch_Critical"
  Constant6/1 -> Data Type Conversion2/1  "Eng_Torque_Mismch_Limp"
  Constant5/1 -> Data Type Conversion1/1  "Eng_Torque_Mismch_Degrad"
  Data Type Conversion/1 -> Bus Creator/1  "Eng_Torque_Mismch_Critical"
  Data Type Conversion1/1 -> Bus Creator/2  "Eng_Torque_Mismch_Degrad"
  Data Type Conversion2/1 -> Bus Creator/3  "Eng_Torque_Mismch_Limp"

== system Clutchless_P2_Parallel_ETE/Clutchless_HSC_ETE/HSC/Camaro Fault Detection/Input Conversions/BMS_Conversions/Override  BMS_gdf 0_1 ==
  note: Override Switch Subsystem
  note: This subsystem is used to override the model value of a signal to a constant value
  In1 : Inport
  Multiport Switch : MultiPortSwitch  DataPortOrder=Zero-based contiguous  Inputs=2  zeroidx=on
  Override Value : Constant  Value=0  OutDataTypeStr=double
  Signal Override Switch 0 = Use Model 1 = Use Constant : Constant
  Out1 : Outport
  wires:
  Override Value/1 -> Multiport Switch/3
  Multiport Switch/1 -> Out1/1
  In1/1 -> Multiport Switch/2
  Signal Override Switch 0 = Use Model 1 = Use Constant/1 -> Multiport Switch/1

== system Clutchless_P2_Parallel_ETE/Clutchless_HSC_ETE/HSC/Camaro Fault Detection/Input Conversions/BMS_Conversions/Override  closeContactorsCmd ==
  note: This subsystem is used to override the model value of a signal to a constant value
  note: Override Switch Subsystem
  In1 : Inport
  Multiport Switch : MultiPortSwitch  DataPortOrder=Zero-based contiguous  Inputs=2  zeroidx=on
  Override Value : Constant  Value=0  OutDataTypeStr=double
  Signal Override Switch 0 = Use Model 1 = Use Constant : Constant  Value=0
  Out1 : Outport
  wires:
  Signal Override Switch 0 = Use Model 1 = Use Constant/1 -> Multiport Switch/1
  In1/1 -> Multiport Switch/2
  Multiport Switch/1 -> Out1/1
  Override Value/1 -> Multiport Switch/3

== system Clutchless_P2_Parallel_ETE/Clutchless_HSC_ETE/HSC/Camaro Fault Detection/Input Conversions/BMS_Conversions/Override  contactorsClsd ==
  note: This subsystem is used to override the model value of a signal to a constant value
  note: Override Switch Subsystem
  In1 : Inport
  Multiport Switch : MultiPortSwitch  DataPortOrder=Zero-based contiguous  Inputs=2  zeroidx=on
  Override Value : Constant  Value=0  OutDataTypeStr=double
  Signal Override Switch 0 = Use Model 1 = Use Constant : Constant  Value=0
  Out1 : Outport
  wires:
  Signal Override Switch 0 = Use Model 1 = Use Constant/1 -> Multiport Switch/1
  In1/1 -> Multiport Switch/2
  Multiport Switch/1 -> Out1/1
  Override Value/1 -> Multiport Switch/3

== system Clutchless_P2_Parallel_ETE/Clutchless_HSC_ETE/HSC/Camaro Fault Detection/Input Conversions/BMS_Conversions/Override  essCur_A ==
  note: Override Switch Subsystem
  note: This subsystem is used to override the model value of a signal to a constant value
  In1 : Inport
  Multiport Switch : MultiPortSwitch  DataPortOrder=Zero-based contiguous  Inputs=2  zeroidx=on
  Override Value : Constant  Value=0  OutDataTypeStr=double
  Signal Override Switch 0 = Use Model 1 = Use Constant : Constant  Value=0
  Out1 : Outport
  wires:
  Override Value/1 -> Multiport Switch/3
  Multiport Switch/1 -> Out1/1
  In1/1 -> Multiport Switch/2
  Signal Override Switch 0 = Use Model 1 = Use Constant/1 -> Multiport Switch/1

== system Clutchless_P2_Parallel_ETE/Clutchless_HSC_ETE/HSC/Camaro Fault Detection/Input Conversions/BMS_Conversions/Override  essSOC_0_1 ==
  note: This subsystem is used to override the model value of a signal to a constant value
  note: Override Switch Subsystem
  In1 : Inport
  Multiport Switch : MultiPortSwitch  DataPortOrder=Zero-based contiguous  Inputs=2  zeroidx=on
  Override Value : Constant  Value=0  OutDataTypeStr=double
  Signal Override Switch 0 = Use Model 1 = Use Constant : Constant  Value=0
  Out1 : Outport
  wires:
  Signal Override Switch 0 = Use Model 1 = Use Constant/1 -> Multiport Switch/1
  In1/1 -> Multiport Switch/2
  Multiport Switch/1 -> Out1/1
  Override Value/1 -> Multiport Switch/3

== system Clutchless_P2_Parallel_ETE/Clutchless_HSC_ETE/HSC/Camaro Fault Detection/Input Conversions/BMS_Conversions/Override  essTemp_C ==
  note: This subsystem is used to override the model value of a signal to a constant value
  note: Override Switch Subsystem
  In1 : Inport
  Multiport Switch : MultiPortSwitch  DataPortOrder=Zero-based contiguous  Inputs=2  zeroidx=on
  Override Value : Constant  Value=0  OutDataTypeStr=double
  Signal Override Switch 0 = Use Model 1 = Use Constant : Constant
  Out1 : Outport
  wires:
  Signal Override Switch 0 = Use Model 1 = Use Constant/1 -> Multiport Switch/1
  In1/1 -> Multiport Switch/2
  Multiport Switch/1 -> Out1/1
  Override Value/1 -> Multiport Switch/3

== system Clutchless_P2_Parallel_ETE/Clutchless_HSC_ETE/HSC/Camaro Fault Detection/Input Conversions/BMS_Conversions/Override  hvBattVolt_V ==
  note: This subsystem is used to override the model value of a signal to a constant value
  note: Override Switch Subsystem
  In1 : Inport
  Multiport Switch : MultiPortSwitch  DataPortOrder=Zero-based contiguous  Inputs=2  zeroidx=on
  Override Value : Constant  Value=0  OutDataTypeStr=double
  Signal Override Switch 0 = Use Model 1 = Use Constant : Constant  Value=0
  Out1 : Outport
  wires:
  Signal Override Switch 0 = Use Model 1 = Use Constant/1 -> Multiport Switch/1
  In1/1 -> Multiport Switch/2
  Multiport Switch/1 -> Out1/1
  Override Value/1 -> Multiport Switch/3

== system Clutchless_P2_Parallel_ETE/Clutchless_HSC_ETE/HSC/Camaro Fault Detection/Input Conversions/BMS_Conversions/Override  hvBusVolt_V ==
  note: Override Switch Subsystem
  note: This subsystem is used to override the model value of a signal to a constant value
  In1 : Inport
  Multiport Switch : MultiPortSwitch  DataPortOrder=Zero-based contiguous  Inputs=2  zeroidx=on
  Override Value : Constant  Value=0  OutDataTypeStr=double
  Signal Override Switch 0 = Use Model 1 = Use Constant : Constant  Value=0
  Out1 : Outport
  wires:
  Override Value/1 -> Multiport Switch/3
  Multiport Switch/1 -> Out1/1
  In1/1 -> Multiport Switch/2
  Signal Override Switch 0 = Use Model 1 = Use Constant/1 -> Multiport Switch/1

== system Clutchless_P2_Parallel_ETE/Clutchless_HSC_ETE/HSC/Camaro Fault Detection/Input Conversions/BMS_Conversions/Override  rollingAliveCnt [1_3] ==
  note: Override Switch Subsystem
  note: This subsystem is used to override the model value of a signal to a constant value
  In1 : Inport
  Multiport Switch : MultiPortSwitch  DataPortOrder=Zero-based contiguous  Inputs=2  zeroidx=on
  Override Value : Constant  Value=0  OutDataTypeStr=double
  Signal Override Switch 0 = Use Model 1 = Use Constant : Constant  Value=0
  Out1 : Outport
  wires:
  Override Value/1 -> Multiport Switch/3
  Multiport Switch/1 -> Out1/1
  In1/1 -> Multiport Switch/2
  Signal Override Switch 0 = Use Model 1 = Use Constant/1 -> Multiport Switch/1

== system Clutchless_P2_Parallel_ETE/Clutchless_HSC_ETE/HSC/Camaro Fault Detection/Input Conversions/BMS_Conversions/Override Fehler_HS_offen ==
  note: This subsystem is used to override the model value of a signal to a constant value
  note: Override Switch Subsystem
  In1 : Inport
  Multiport Switch : MultiPortSwitch  DataPortOrder=Zero-based contiguous  Inputs=2  zeroidx=on
  Override Value : Constant  Value=0  OutDataTypeStr=double
  Signal Override Switch 0 = Use Model 1 = Use Constant : Constant
  Out1 : Outport
  wires:
  Signal Override Switch 0 = Use Model 1 = Use Constant/1 -> Multiport Switch/1
  In1/1 -> Multiport Switch/2
  Multiport Switch/1 -> Out1/1
  Override Value/1 -> Multiport Switch/3

== system Clutchless_P2_Parallel_ETE/Clutchless_HSC_ETE/HSC/Camaro Fault Detection/Input Conversions/BMS_Conversions/Override Fehler_HS_verschweisst ==
  note: Override Switch Subsystem
  note: This subsystem is used to override the model value of a signal to a constant value
  In1 : Inport
  Multiport Switch : MultiPortSwitch  DataPortOrder=Zero-based contiguous  Inputs=2  zeroidx=on
  Override Value : Constant  Value=0  OutDataTypeStr=double
  Signal Override Switch 0 = Use Model 1 = Use Constant : Constant
  Out1 : Outport
  wires:
  Override Value/1 -> Multiport Switch/3
  Multiport Switch/1 -> Out1/1
  In1/1 -> Multiport Switch/2
  Signal Override Switch 0 = Use Model 1 = Use Constant/1 -> Multiport Switch/1

== system Clutchless_P2_Parallel_ETE/Clutchless_HSC_ETE/HSC/Camaro Fault Detection/Input Conversions/DriverInput_Conversions/Override  KeyPos [0_3] ==
  note: Override Switch Subsystem
  note: This subsystem is used to override the model value of a signal to a constant value
  In1 : Inport
  Multiport Switch : MultiPortSwitch  DataPortOrder=Zero-based contiguous  Inputs=2  zeroidx=on
  Override Value : Constant  Value=0  OutDataTypeStr=double
  Signal Override Switch 0 = Use Model 1 = Use Constant : Constant  Value=0
  Out1 : Outport
  wires:
  Override Value/1 -> Multiport Switch/3
  Multiport Switch/1 -> Out1/1
  In1/1 -> Multiport Switch/2
  Signal Override Switch 0 = Use Model 1 = Use Constant/1 -> Multiport Switch/1

== system Clutchless_P2_Parallel_ETE/Clutchless_HSC_ETE/HSC/Camaro Fault Detection/Input Conversions/DriverInput_Conversions/Override APP (%) ==
  note: Override Switch Subsystem
  note: This subsystem is used to override the model value of a signal to a constant value
  In1 : Inport
  Multiport Switch : MultiPortSwitch  DataPortOrder=Zero-based contiguous  Inputs=2  zeroidx=on
  Override Value : Constant  Value=0  OutDataTypeStr=double
  Signal Override Switch 0 = Use Model 1 = Use Constant : Constant  Value=0
  Out1 : Outport
  wires:
  Override Value/1 -> Multiport Switch/3
  Multiport Switch/1 -> Out1/1
  In1/1 -> Multiport Switch/2
  Signal Override Switch 0 = Use Model 1 = Use Constant/1 -> Multiport Switch/1

== system Clutchless_P2_Parallel_ETE/Clutchless_HSC_ETE/HSC/Camaro Fault Detection/Input Conversions/DriverInput_Conversions/Override APP (%)1 ==
  note: This subsystem is used to override the model value of a signal to a constant value
  note: Override Switch Subsystem
  In1 : Inport
  Multiport Switch : MultiPortSwitch  DataPortOrder=Zero-based contiguous  Inputs=2  zeroidx=on
  Override Value : Constant  Value=0  OutDataTypeStr=double
  Signal Override Switch 0 = Use Model 1 = Use Constant : Constant  Value=0
  Out1 : Outport
  wires:
  Signal Override Switch 0 = Use Model 1 = Use Constant/1 -> Multiport Switch/1
  In1/1 -> Multiport Switch/2
  Multiport Switch/1 -> Out1/1
  Override Value/1 -> Multiport Switch/3

== system Clutchless_P2_Parallel_ETE/Clutchless_HSC_ETE/HSC/Camaro Fault Detection/Input Conversions/DriverInput_Conversions/Override BPP (%) ==
  note: This subsystem is used to override the model value of a signal to a constant value
  note: Override Switch Subsystem
  In1 : Inport
  Multiport Switch : MultiPortSwitch  DataPortOrder=Zero-based contiguous  Inputs=2  zeroidx=on
  Override Value : Constant  Value=0  OutDataTypeStr=double
  Signal Override Switch 0 = Use Model 1 = Use Constant : Constant  Value=0
  Out1 : Outport
  wires:
  Signal Override Switch 0 = Use Model 1 = Use Constant/1 -> Multiport Switch/1
  In1/1 -> Multiport Switch/2
  Multiport Switch/1 -> Out1/1
  Override Value/1 -> Multiport Switch/3

== system Clutchless_P2_Parallel_ETE/Clutchless_HSC_ETE/HSC/Camaro Fault Detection/Input Conversions/DriverInput_Conversions/Override PRNDL ==
  note: Override Switch Subsystem
  note: This subsystem is used to override the model value of a signal to a constant value
  In1 : Inport
  Multiport Switch : MultiPortSwitch  DataPortOrder=Zero-based contiguous  Inputs=2  zeroidx=on
  Override Value : Constant  Value=0  OutDataTypeStr=double
  Signal Override Switch 0 = Use Model 1 = Use Constant : Constant  Value=0
  Out1 : Outport
  wires:
  Override Value/1 -> Multiport Switch/3
  Multiport Switch/1 -> Out1/1
  In1/1 -> Multiport Switch/2
  Signal Override Switch 0 = Use Model 1 = Use Constant/1 -> Multiport Switch/1

== system Clutchless_P2_Parallel_ETE/Clutchless_HSC_ETE/HSC/Camaro Fault Detection/Input Conversions/DriverInput_Conversions/Override Regen ==
  note: Override Switch Subsystem
  note: This subsystem is used to override the model value of a signal to a constant value
  In1 : Inport
  Multiport Switch : MultiPortSwitch  DataPortOrder=Zero-based contiguous  Inputs=2  zeroidx=on
  Override Value : Constant  Value=0  OutDataTypeStr=double
  Signal Override Switch 0 = Use Model 1 = Use Constant : Constant  Value=0
  Out1 : Outport
  wires:
  Override Value/1 -> Multiport Switch/3
  Multiport Switch/1 -> Out1/1
  In1/1 -> Multiport Switch/2
  Signal Override Switch 0 = Use Model 1 = Use Constant/1 -> Multiport Switch/1

== system Clutchless_P2_Parallel_ETE/Clutchless_HSC_ETE/HSC/Camaro Fault Detection/Input Conversions/DriverInput_Conversions/Override V [mph] ==
  note: This subsystem is used to override the model value of a signal to a constant value
  note: Override Switch Subsystem
  In1 : Inport
  Multiport Switch : MultiPortSwitch  DataPortOrder=Zero-based contiguous  Inputs=2  zeroidx=on
  Override Value : Constant  Value=0  OutDataTypeStr=double
  Signal Override Switch 0 = Use Model 1 = Use Constant : Constant  Value=0
  Out1 : Outport
  wires:
  Signal Override Switch 0 = Use Model 1 = Use Constant/1 -> Multiport Switch/1
  In1/1 -> Multiport Switch/2
  Multiport Switch/1 -> Out1/1
  Override Value/1 -> Multiport Switch/3

== system Clutchless_P2_Parallel_ETE/Clutchless_HSC_ETE/HSC/Camaro Fault Detection/Input Conversions/ECM_Conversions/Override  ECMTrqCmd_Nm ==
  note: This subsystem is used to override the model value of a signal to a constant value
  note: Override Switch Subsystem
  In1 : Inport
  Multiport Switch : MultiPortSwitch  DataPortOrder=Zero-based contiguous  Inputs=2  zeroidx=on
  Override Value : Constant  Value=0  OutDataTypeStr=double
  Signal Override Switch 0 = Use Model 1 = Use Constant : Constant  Value=0
  Out1 : Outport
  wires:
  Signal Override Switch 0 = Use Model 1 = Use Constant/1 -> Multiport Switch/1
  In1/1 -> Multiport Switch/2
  Multiport Switch/1 -> Out1/1
  Override Value/1 -> Multiport Switch/3

== system Clutchless_P2_Parallel_ETE/Clutchless_HSC_ETE/HSC/Camaro Fault Detection/Input Conversions/ECM_Conversions/Override  ECMrollingAliveCnt ==
  note: Override Switch Subsystem
  note: This subsystem is used to override the model value of a signal to a constant value
  In1 : Inport
  Multiport Switch : MultiPortSwitch  DataPortOrder=Zero-based contiguous  Inputs=2  zeroidx=on
  Override Value : Constant  Value=0  OutDataTypeStr=double
  Signal Override Switch 0 = Use Model 1 = Use Constant : Constant  Value=0
  Out1 : Outport
  wires:
  Override Value/1 -> Multiport Switch/3
  Multiport Switch/1 -> Out1/1
  In1/1 -> Multiport Switch/2
  Signal Override Switch 0 = Use Model 1 = Use Constant/1 -> Multiport Switch/1

== system Clutchless_P2_Parallel_ETE/Clutchless_HSC_ETE/HSC/Camaro Fault Detection/Input Conversions/ECM_Conversions/Override  EngActStdyStTorq_Nm ==
  note: Override Switch Subsystem
  note: This subsystem is used to override the model value of a signal to a constant value
  In1 : Inport
  Multiport Switch : MultiPortSwitch  DataPortOrder=Zero-based contiguous  Inputs=2  zeroidx=on
  Override Value : Constant  Value=0  OutDataTypeStr=double
  Signal Override Switch 0 = Use Model 1 = Use Constant : Constant  Value=0
  Out1 : Outport
  wires:
  Override Value/1 -> Multiport Switch/3
  Multiport Switch/1 -> Out1/1
  In1/1 -> Multiport Switch/2
  Signal Override Switch 0 = Use Model 1 = Use Constant/1 -> Multiport Switch/1

== system Clutchless_P2_Parallel_ETE/Clutchless_HSC_ETE/HSC/Camaro Fault Detection/Input Conversions/ECM_Conversions/Override  EngRunAtv ==
  note: This subsystem is used to override the model value of a signal to a constant value
  note: Override Switch Subsystem
  In1 : Inport
  Multiport Switch : MultiPortSwitch  DataPortOrder=Zero-based contiguous  Inputs=2  zeroidx=on
  Override Value : Constant  Value=0  OutDataTypeStr=double
  Signal Override Switch 0 = Use Model 1 = Use Constant : Constant  Value=0
  Out1 : Outport
  wires:
  Signal Override Switch 0 = Use Model 1 = Use Constant/1 -> Multiport Switch/1
  In1/1 -> Multiport Switch/2
  Multiport Switch/1 -> Out1/1
  Override Value/1 -> Multiport Switch/3

== system Clutchless_P2_Parallel_ETE/Clutchless_HSC_ETE/HSC/Camaro Fault Detection/Input Conversions/ECM_Conversions/Override  EngineSpeed_rpm ==
  note: This subsystem is used to override the model value of a signal to a constant value
  note: Override Switch Subsystem
  In1 : Inport
  Multiport Switch : MultiPortSwitch  DataPortOrder=Zero-based contiguous  Inputs=2  zeroidx=on
  Override Value : Constant  Value=0  OutDataTypeStr=double
  Signal Override Switch 0 = Use Model 1 = Use Constant : Constant  Value=0
  Out1 : Outport
  wires:
  Signal Override Switch 0 = Use Model 1 = Use Constant/1 -> Multiport Switch/1
  In1/1 -> Multiport Switch/2
  Multiport Switch/1 -> Out1/1
  Override Value/1 -> Multiport Switch/3

== system Clutchless_P2_Parallel_ETE/Clutchless_HSC_ETE/HSC/Camaro Fault Detection/Input Conversions/ECM_Conversions/Override  Engine_Temp[DegC] ==
  note: Override Switch Subsystem
  note: This subsystem is used to override the model value of a signal to a constant value
  In1 : Inport
  Multiport Switch : MultiPortSwitch  DataPortOrder=Zero-based contiguous  Inputs=2  zeroidx=on
  Override Value : Constant  Value=0  OutDataTypeStr=double
  Signal Override Switch 0 = Use Model 1 = Use Constant : Constant  Value=0
  Out1 : Outport
  wires:
  Override Value/1 -> Multiport Switch/3
  Multiport Switch/1 -> Out1/1
  In1/1 -> Multiport Switch/2
  Signal Override Switch 0 = Use Model 1 = Use Constant/1 -> Multiport Switch/1

== system Clutchless_P2_Parallel_ETE/Clutchless_HSC_ETE/HSC/Camaro Fault Detection/Input Conversions/TCM_Conversions/Override  LockupCmd ==
  note: This subsystem is used to override the model value of a signal to a constant value
  note: Override Switch Subsystem
  In1 : Inport
  Multiport Switch : MultiPortSwitch  DataPortOrder=Zero-based contiguous  Inputs=2  zeroidx=on
  Override Value : Constant  Value=0  OutDataTypeStr=double
  Signal Override Switch 0 = Use Model 1 = Use Constant : Constant  Value=0
  Out1 : Outport
  wires:
  Signal Override Switch 0 = Use Model 1 = Use Constant/1 -> Multiport Switch/1
  In1/1 -> Multiport Switch/2
  Multiport Switch/1 -> Out1/1
  Override Value/1 -> Multiport Switch/3

== system Clutchless_P2_Parallel_ETE/Clutchless_HSC_ETE/HSC/Camaro Fault Detection/Input Conversions/TCM_Conversions/Override  LvrPosTrnsShft  ==
  note: This subsystem is used to override the model value of a signal to a constant value
  note: Override Switch Subsystem
  In1 : Inport
  Multiport Switch : MultiPortSwitch  DataPortOrder=Zero-based contiguous  Inputs=2  zeroidx=on
  Override Value : Constant  Value=0  OutDataTypeStr=double
  Signal Override Switch 0 = Use Model 1 = Use Constant : Constant  Value=0
  Out1 : Outport
  wires:
  Signal Override Switch 0 = Use Model 1 = Use Constant/1 -> Multiport Switch/1
  In1/1 -> Multiport Switch/2
  Multiport Switch/1 -> Out1/1
  Override Value/1 -> Multiport Switch/3

== system Clutchless_P2_Parallel_ETE/Clutchless_HSC_ETE/HSC/Camaro Fault Detection/Input Conversions/TCM_Conversions/Override  TransEstGear ==
  note: This subsystem is used to override the model value of a signal to a constant value
  note: Override Switch Subsystem
  In1 : Inport
  Multiport Switch : MultiPortSwitch  DataPortOrder=Zero-based contiguous  Inputs=2  zeroidx=on
  Override Value : Constant  Value=0  OutDataTypeStr=double
  Signal Override Switch 0 = Use Model 1 = Use Constant : Constant  Value=0
  Out1 : Outport
  wires:
  Signal Override Switch 0 = Use Model 1 = Use Constant/1 -> Multiport Switch/1
  In1/1 -> Multiport Switch/2
  Multiport Switch/1 -> Out1/1
  Override Value/1 -> Multiport Switch/3

== system Clutchless_P2_Parallel_ETE/Clutchless_HSC_ETE/HSC/Camaro Fault Detection/Input Conversions/TCM_Conversions/Override  rollingAliveCnt [123] ==
  note: This subsystem is used to override the model value of a signal to a constant value
  note: Override Switch Subsystem
  In1 : Inport
  Multiport Switch : MultiPortSwitch  DataPortOrder=Zero-based contiguous  Inputs=2  zeroidx=on
  Override Value : Constant  Value=0  OutDataTypeStr=double
  Signal Override Switch 0 = Use Model 1 = Use Constant : Constant  Value=0
  Out1 : Outport
  wires:
  Signal Override Switch 0 = Use Model 1 = Use Constant/1 -> Multiport Switch/1
  In1/1 -> Multiport Switch/2
  Multiport Switch/1 -> Out1/1
  Override Value/1 -> Multiport Switch/3

== system Clutchless_P2_Parallel_ETE/Clutchless_HSC_ETE/HSC/Camaro Fault Detection/Input Conversions/TCM_Conversions/TCM_RollinAliveCounter ==
  Constant : Constant  Value=0
  Constant8 : Constant
  Rolling Alive Counter1 : Stateflow chart  TreatAsAtomicUnit=on
  Switch1 : Switch  Criteria=u2 > Threshold
  Out1 : Outport
  wires:
  Constant/1 -> [TCM_CAN_fault]
  Switch1/1 -> Out1/1  "TCMRollingAliveCnt [0 1 2 3]"
  [TCM_CAN_fault] -> Switch1/2
  Rolling Alive Counter1/1(RollingAliveCnt) -> Switch1/3
  Constant8/1 -> Switch1/1

== system Clutchless_P2_Parallel_ETE/Clutchless_HSC_ETE/HSC/Camaro Fault Detection/Signal Diagnostic/Driver Signal Diagnostic/APP_Crosscheck ==
  In1 : Inport
  In2 : Inport  Port=2
  Abs : Abs
  Compare To Constant : simulink/Logic and Bit Operations/Compare To Constant  relop=<=  const=0.5  OutDataTypeStr=boolean
  Sum : Sum  Inputs=+-
  Out1 : Outport
  wires:
  Sum/1 -> Abs/1
  Abs/1 -> Compare To Constant/1
  In1/1 -> Sum/1
  In2/1 -> Sum/2
  Compare To Constant/1 -> Out1/1  "Drv_APP_Agree"
